simulink model "EC_control_harness"  (R2023b)
settings: Solver=FixedStepAuto  StartTime=0.0  StopTime=inf  FixedStep=2.6667e-04  RelTol=1e-4  AbsTol=1e-6
settings Model: DataDictionary=fmuGenerationDictionay.sldd  ModifiedByFormat=Third Equation Ltd  Creator=Third Equation Ltd  LastModifiedBy=Third Equation Ltd
settings ConfigSet: Description=|
  | Reference configuration for protected model and FMU generation
  | Sample frequency = 3750 Hz
settings SolverCC: AutoScaleAbsTol=off  AlgebraicLoopSolver=TrustRegion  MaxZcPerStep=1
settings DataIOCC: ExternalInput=[]  InitialState=[]  SaveFormat=Array  SaveOutput=off  SaveTime=off  ReturnWorkspaceOutputs=off
settings OptimizationCC: BlockReduction=off  BooleanDataType=off  ReuseModelBlockBuffer=off  ExpressionDepthLimit=2147483647  InitFltsAndDblsToZero=on
settings DebuggingCC: SaveWithParameterizedLinksMsg=none  SignalResolutionControl=TryResolveAllWithWarning  MultiTaskDSMMsg=warning  MultiTaskCondExecSysMsg=none  IntegerOverflowMsg=none  FcnCallInpInsideContextMsg=warning  UnconnectedInputMsg=warning  UnconnectedOutputMsg=warning  UnconnectedLineMsg=warning  StateNameClashWarn=warning  SFUnexpectedBacktrackingDiag=warning  SFNoUnconditionalDefaultTransitionDiag=warning  SFExecutionAtInitializationDiag=none  IntegerSaturationMsg=none  UnderSpecifiedDimensionMsg=warning  ArithmeticOperatorsInVariantConditions=warning
settings HardwareCC: ProdBitPerPointer=32  ProdBitPerSizeT=32  ProdBitPerPtrDiffT=32  ProdLargestAtomicFloat=None  ProdWordSize=32  ProdHWDeviceType=Custom Processor->Custom Processor
settings ModelReferenceCC: EnableRefExpFcnMdlSchedulingChecks=on  PropagateSignalLabelsOutOfModel=off
settings SFSimCC: SimUseLocalCustomCode=off  CustomCodeUndefinedFunction=UseInterfaceOnly
settings RTWCC: Description=FMU2CS  SystemTargetFile=fmu2cs.tlc  TemplateMakefile=fmu2cs_default_tmf  RTWUseLocalCustomCode=off  DLArmComputeVersion=19.05
settings CodeAppCC: StateflowObjectComments=on
settings GRTTargetCC: TargetLangStandard=C89/C90 (ANSI)  CombineOutputUpdateFcns=off  MatFileLogging=off
settings ConfigComp: CovMetricSettings=dw  CovSaveCumulativeToWorkspaceVar=on  CovSaveSingleToWorkspaceVar=on  CovExternalEMLEnable=off  CovSFcnEnable=off

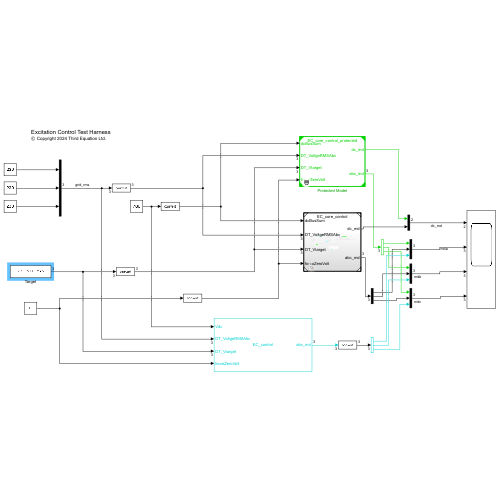
[thumbnail: Simulink's stored preview of the top-level diagram]
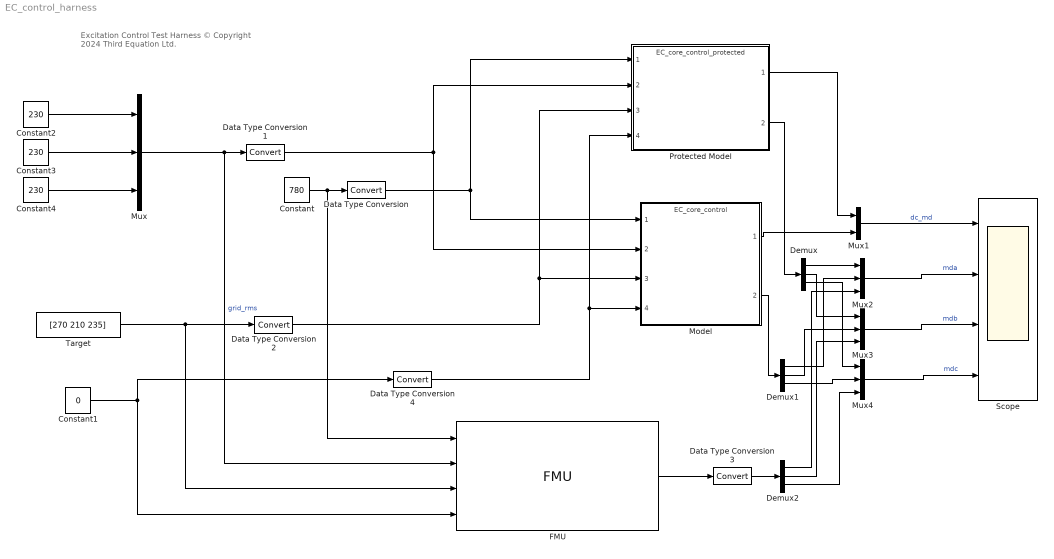
== system EC_control_harness ==
  note: Excitation Control Test Harness
      | © Copyright 2024 Third Equation Ltd.
  Constant : Constant  Value=780
  Constant1 : Constant  Value=0  OutDataTypeStr=int32
  Constant2 : Constant  Value=230
  Constant3 : Constant  Value=230
  Constant4 : Constant  Value=230
  Data Type Conversion{,1..4} (5 alike) : DataTypeConversion  SaturateOnIntegerOverflow=off  RndMeth=Floor
  Demux : Demux  Outputs=3
  Demux1 : Demux  Outputs=3
  Demux2 : Demux  Outputs=3
  FMU : FMU  FMUName=EC_control.fmu  FMUMode=CoSimulation  FMUCreateBusObject=off  FMUInitializeEnumObject=off  FMUCachedDialogLayout="{\"Geometry\":[-1314,614,433,389],\"ParameterColumnsWidthConfig\":\"{\\\"columns\\\":[{\\\"name\\\":\\\"Parameter\\\",\\\"width\\\":181},{\\\"name\\\":\\\"Value\\\",\\\"width\\\":145},{\\\"name\\\":\\\"Unit\\\",\\\"width\\\":135},{\\\"name\\\":\\\"Description\\\",\\\"width\\\":190}]}\",\"InputColumnsWidthConfig\":\"{\\\"columns\\\":[{\\\"name\\\":\\\"Name\\\",\\\"width\\\":111},{\\\"name\\\":\\\"Visibility\\\",\\\"width\\\":60},{\\\"name\\\":\\\"Start\\\",\\\"width\\\":103},{\\\"name\\\":\\\"Unit\\\",\\\"width\\\":99},{\\\"name\\\":\\\"Type Object\\\",\\\"width\\\":144}]}\",\"OutputColumnsWidthConfig\":\"{\\\"columns\\\":[{\\\"name\\\":\\\"Name\\\",\\\"width\\\":111},{\\\"name\\\":\\\"Visibility\\\",\\\"width\\\":60},{\\\"name\\\":\\\"Start\\\",\\\"width\\\":103},{\\\"name\\\":\\\"Unit\\\",\\\"width\\\":99},{\\\"name\\\":\\\"Type Object\\\",\\\"width\\\":144}]}\"}"
      mask Type: EC_control [Co-Simulation, v2.0]
      mask Display:
      | if (exist([Simulink.fileGenControl('get','CacheFolder') '\slprj\_fmu\25bc88b116eb2d6cca0888ab3059811e\EC_control\model.png'],'file'))
      |     image([Simulink.fileGenControl('get','CacheFolder') '\slprj\_fmu\25bc88b116eb2d6cca0888ab3059811e\EC_control\model.png']);
      | else
      |     disp('EC_control');
      | end
      | port_label('output',1,'abc_md');
      | port_label('input',1,'Vdc');
      | port_label('input',2,'DT_VoltgeRMSAbc');
      | port_label('input',3,'DT_Vtarget');
      | port_label('input',4,'forceZeroVolt');
  Model : ModelReference  ModelNameDialog=EC_core_control.slx  SimulationMode=Normal  ModelReferenceVersion=1.40
  Mux{,2..4} (4 alike) : Mux  Inputs=3
  Mux1 : Mux  Inputs=2
  Protected Model : ModelReference  ModelNameDialog=EC_core_control_protected.slxp  ModelReferenceVersion=1.40  CopyOfModelProtected=on
  Scope : Scope  NumInputPorts=4
  Target : Constant  Value=[270 210 235]
  wires:
  Constant4/1 -> Mux/3
  Constant3/1 -> Mux/2
  Target/1 -> FMU/3, Data Type Conversion2/1
  Mux/1 -> FMU/2, Data Type Conversion1/1  "grid_rms"
  Constant2/1 -> Mux/1
  Constant/1 -> FMU/1, Data Type Conversion/1
  Data Type Conversion/1 -> Model/1, Protected Model/1
  Mux2/1 -> Scope/2  "mda"
  Mux1/1 -> Scope/1  "dc_md"
  Model/1 -> Mux1/2
  Protected Model/2 -> Demux/1
  Protected Model/1 -> Mux1/1
  Mux3/1 -> Scope/3  "mdb"
  Mux4/1 -> Scope/4  "mdc"
  Model/2 -> Demux1/1
  Demux/1 -> Mux2/1
  Demux/2 -> Mux3/1
  Demux/3 -> Mux4/1
  Demux1/1 -> Mux2/2
  Demux1/2 -> Mux3/2
  Demux1/3 -> Mux4/2
  FMU/1 -> Data Type Conversion3/1
  Demux2/1 -> Mux2/3
  Demux2/2 -> Mux3/3
  Demux2/3 -> Mux4/3
  Data Type Conversion3/1 -> Demux2/1
  Data Type Conversion1/1 -> Model/2, Protected Model/2
  Data Type Conversion2/1 -> Model/3, Protected Model/3
  Constant1/1 -> FMU/4, Data Type Conversion4/1
  Data Type Conversion4/1 -> Protected Model/4, Model/4
